simulink model "simulate_H_inf_state"  (R2013b)
settings: Solver=ode8  StartTime=0.0  StopTime=40  FixedStep=T_s  MaxStep=Auto  MinStep=Auto  RelTol=1e-3
values from neighbouring files (symbols this model uses):
  A = [0 0                                                1 0 ... (first row only)    [H_inf_state_feedback.m]    (also in Hinf_discrete_state_feedback_control (Dogan Onur ARISOY's conflicted copy 2017-02-06).m = a; Hinf_discrete_state_feedback_control.m = a; Hinf_discrete_state_feedback_control_ceyrek_tasit.m = a; bina_sistem.m = [zeros(4,4)         eye(4))
  Ac = [-1.01887           0.90506           -0.00215 ... (first row only)    [Hinf_discrete_state_feedback_control (Dogan Onur ARISOY's conflicted copy 2017-02-06).m]    (also in Hinf_discrete_state_feedback_control.m = [zeros(2) eye(2); Hinf_discrete_state_feedback_control_ceyrek_tasit.m = [0 0 1 0; LMI_Dynamic_Output.m = value(Ac); bench__lmi_state_hinf.m = [zeros(4) eye(4))
  B1 = [0;0;0;k2/m2]    [H_inf_state_feedback.m]    (also in Hinf_discrete_state_feedback_control (Dogan Onur ARISOY's conflicted copy 2017-02-06).m = b(:,1:size(Bc1,2)); Hinf_discrete_state_feedback_control.m = b(:,1:size(Bc1,2)); Hinf_discrete_state_feedback_control_ceyrek_tasit.m = b(:,1:size(Bc1,2)); bina_sistem.m = zeros(8,2))
  Bc1 = [0 ... (first row only)    [Hinf_discrete_state_feedback_control (Dogan Onur ARISOY's conflicted copy 2017-02-06).m]    (also in Hinf_discrete_state_feedback_control.m = [0;0;0;k2/m2]; Hinf_discrete_state_feedback_control_ceyrek_tasit.m = [0;0;0;k2/m2]; bench__lmi_state_hinf.m = zeros(8,2); bina__lmi_state_hinf.m = zeros(size(Ac,1),2))
  Bc2 = [1 ... (first row only)    [Hinf_discrete_state_feedback_control (Dogan Onur ARISOY's conflicted copy 2017-02-06).m]    (also in Hinf_discrete_state_feedback_control.m = [0;0;1/m1;-1/m2]; Hinf_discrete_state_feedback_control_ceyrek_tasit.m = [0;0;1/m1;-1/m2]; bench__lmi_state_hinf.m = [zeros(4,1);-1/m1;1/m2;0;0]; bina__lmi_state_hinf.m = [zeros(size(M,1),1);-1/m1;1/m2;zeros(size(M,1)-2,1)])
  C = c(1:size(Cc1,1),:)    [Hinf_discrete_state_feedback_control (Dogan Onur ARISOY's conflicted copy 2017-02-06).m]    (also in Hinf_discrete_state_feedback_control.m; Hinf_discrete_state_feedback_control_ceyrek_tasit.m; bina_sistem.m = [c1+c2          -c2              0             0; dis_state_space.m)
  Cc1 = [1  0 0 ... (first row only)    [Hinf_discrete_state_feedback_control (Dogan Onur ARISOY's conflicted copy 2017-02-06).m]    (also in Hinf_discrete_state_feedback_control.m = [1 0 0 0; Hinf_discrete_state_feedback_control_ceyrek_tasit.m = [1 0 0 0;0 1 0 0]; bench__lmi_state_hinf.m = [eye(8)]; bina__lmi_state_hinf.m = [eye(size(Ac,1))])
  E1 = b(:,size(Bc1,2)+1:size(b,2))    [Hinf_discrete_state_feedback_control (Dogan Onur ARISOY's conflicted copy 2017-02-06).m]    (also in Hinf_discrete_state_feedback_control.m; Hinf_discrete_state_feedback_control_ceyrek_tasit.m; dis_state_space.m = b(:,1:size(Bc1,2)); dynamic_output_control.mat = [0.0712527170191 0.000860589552497 4.20229137535e-06 1.11081)
  Kc = LMI_state(Ac,Bc1,Bc2,Cc1,Dc11,Dc12)    [bench__lmi_state_hinf.m]    (also in bina__lmi_state_hinf.m; dynamic_output_control.mat = [22567.2871292 -274430.071266 372104.006554 -47167.8566337 8; lmi_state_hinf.m)
  Kd = Y*Q^-1    [Hinf_discrete_state_feedback_control.m]    (also in bench__lmi_state_hinf.m = LMI_state_dis(A,B1,E1,C,B2,E2); bina__lmi_state_hinf.m = LMI_state_dis(A,B1,E1,C,B2,E2); dynamic_output_control.mat = [-308144.446712 -160117.916012 305677.057837 174380.125501 7; lmi_state_hinf.m = LMI_state_dis(A,B1,E1,C,B2,E2))
  T_s = 1e-6    (= 1e-06)    [Hinf_discrete_state_feedback_control (Dogan Onur ARISOY's conflicted copy 2017-02-06).m]    (also in Hinf_discrete_state_feedback_control.m = 0.0001; Hinf_discrete_state_feedback_control_ceyrek_tasit.m = 0.01; bench__lmi_state_hinf.m = 0.01; bina__lmi_state_hinf.m = 0.01)
settings Model: Creator=mert  LastModifiedBy=oguzhan
settings SolverCC: InitialStep=Auto
settings DebuggingCC: StateNameClashWarn=warning

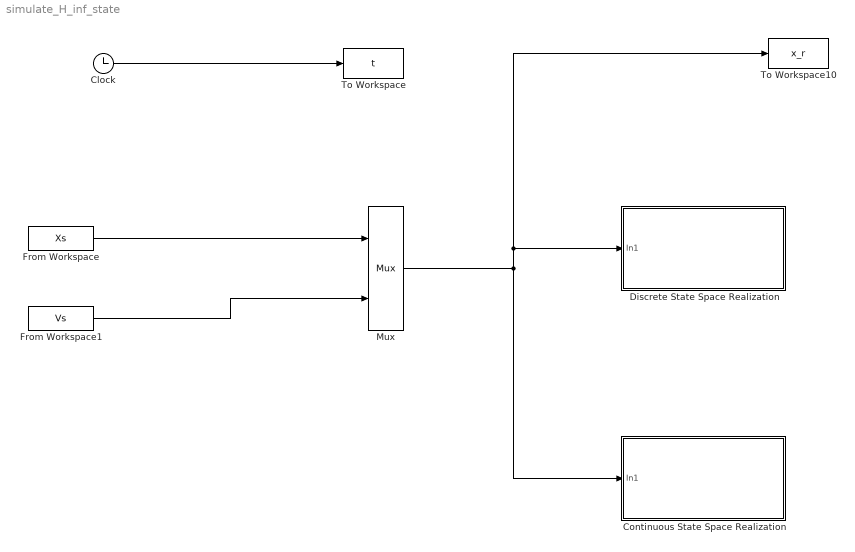
== system simulate_H_inf_state ==
  Clock : Clock
  Continuous State Space Realization : Subsystem
  Discrete State Space Realization : Subsystem
  From Workspace : FromWorkspace  VariableName=Xs
  From Workspace1 : FromWorkspace  VariableName=Vs
  Mux : Mux  Inputs=2
  To Workspace : ToWorkspace  VariableName=t  SampleTime=-1
  To Workspace10 : ToWorkspace  VariableName=x_r  SampleTime=-1
  wires:
  From Workspace/1 -> Mux/1
  From Workspace1/1 -> Mux/2
  Clock/1 -> To Workspace/1
  Mux/1 -> Continuous State Space Realization/1(In1), To Workspace10/1, Discrete State Space Realization/1(In1)

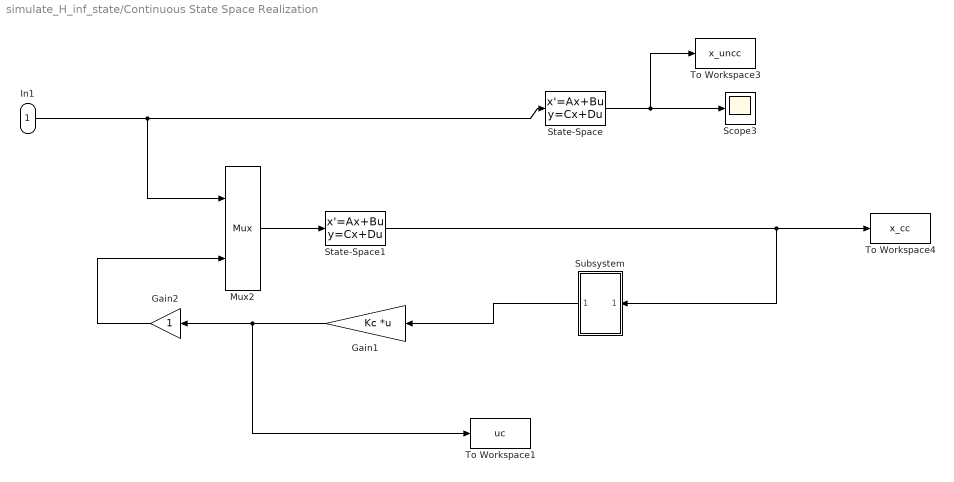
== system simulate_H_inf_state/Continuous State Space Realization ==
  In1 : Inport
  Gain1 : Gain  Gain=Kc  Multiplication=Matrix(K*u) (u vector)
  Gain2 : Gain
  Mux2 : Mux  Inputs=2
  Scope3 : Scope
      settings: SaveName=ScopeData3
  State-Space : StateSpace  A=Ac  B=Bc1  C=[Cc1;Ac(7:12,:)]  D=[zeros(size(Cc1,1),size(Bc1,2));Bc1(7:12,:)]  X0=0
  State-Space1 : StateSpace  A=Ac  B=[Bc1 Bc2]  C=[Cc1;Ac(7:12,:)]  D=[zeros(size(Cc1,1),size([Bc1 Bc2],2));[Bc1(7:12,:) Bc2(7:12,:)]]  X0=0
  Subsystem : Subsystem
  To Workspace1 : ToWorkspace  VariableName=uc  SampleTime=-1
  To Workspace3 : ToWorkspace  VariableName=x_uncc  SampleTime=-1  SaveFormat=Structure
  To Workspace4 : ToWorkspace  VariableName=x_cc  SampleTime=-1  SaveFormat=Structure
  wires:
  State-Space/1 -> To Workspace3/1, Scope3/1
  State-Space1/1 -> Subsystem/1(In1), To Workspace4/1
  Mux2/1 -> State-Space1/1
  In1/1 -> State-Space/1, Mux2/1
  Gain2/1 -> Mux2/2
  Gain1/1 -> To Workspace1/1, Gain2/1
  Subsystem/1(Out1) -> Gain1/1

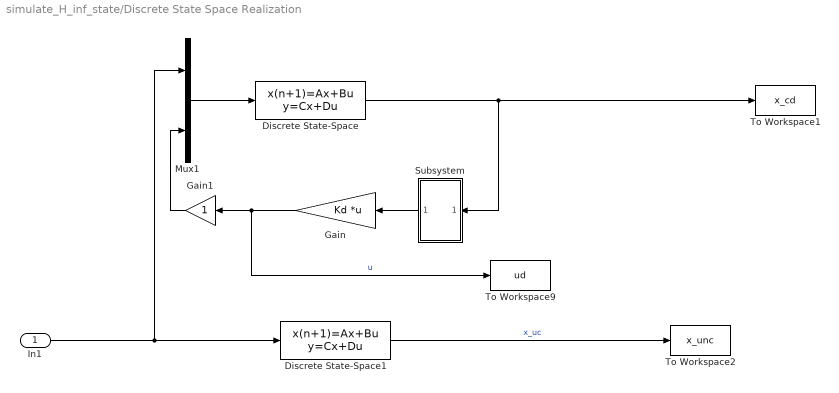
== system simulate_H_inf_state/Discrete State Space Realization ==
  In1 : Inport
  Discrete State-Space : DiscreteStateSpace  A=A  B=[E1 B1]  C=[C; A(7:12,:)]  D=[zeros(size(C,1),size([E1 B1],2));[E1(7:12,:) B1(7:12,:)]]  SampleTime=T_s
  Discrete State-Space1 : DiscreteStateSpace  A=A  B=E1  C=[C;A(7:12,:)]  D=[zeros(size(C,1),size(E1,2));E1(7:12,:)]  SampleTime=T_s
  Gain : Gain  Gain=Kd  Multiplication=Matrix(K*u) (u vector)
  Gain1 : Gain
  Mux1 : Mux  Inputs=2
  Subsystem : Subsystem
  To Workspace1 : ToWorkspace  VariableName=x_cd  SampleTime=-1  SaveFormat=Structure
  To Workspace2 : ToWorkspace  VariableName=x_unc  SampleTime=-1  SaveFormat=Structure
  To Workspace9 : ToWorkspace  VariableName=ud  SampleTime=-1
  wires:
  In1/1 -> Discrete State-Space1/1, Mux1/1
  Gain/1 -> To Workspace9/1, Gain1/1  "u"
  Discrete State-Space1/1 -> To Workspace2/1  "x_uc"
  Mux1/1 -> Discrete State-Space/1
  Discrete State-Space/1 -> To Workspace1/1, Subsystem/1(In1)
  Gain1/1 -> Mux1/2
  Subsystem/1(Out1) -> Gain/1

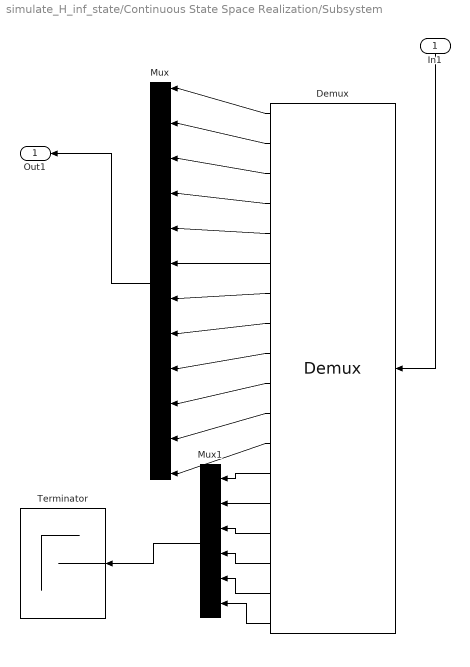
== system simulate_H_inf_state/Continuous State Space Realization/Subsystem ==
  In1 : Inport
  Demux : Demux  Outputs=18
  Mux : Mux  Inputs=12
  Mux1 : Mux  Inputs=6
  Terminator : Terminator
  Out1 : Outport
  wires:
  Mux/1 -> Out1/1
  Demux/2 -> Mux/2
  In1/1 -> Demux/1
  Demux/1 -> Mux/1
  Demux/3 -> Mux/3
  Demux/4 -> Mux/4
  Demux/5 -> Mux/5
  Demux/6 -> Mux/6
  Demux/7 -> Mux/7
  Demux/8 -> Mux/8
  Demux/9 -> Mux/9
  Demux/10 -> Mux/10
  Demux/11 -> Mux/11
  Demux/12 -> Mux/12
  Demux/13 -> Mux1/1
  Demux/14 -> Mux1/2
  Demux/15 -> Mux1/3
  Demux/16 -> Mux1/4
  Demux/17 -> Mux1/5
  Demux/18 -> Mux1/6
  Mux1/1 -> Terminator/1

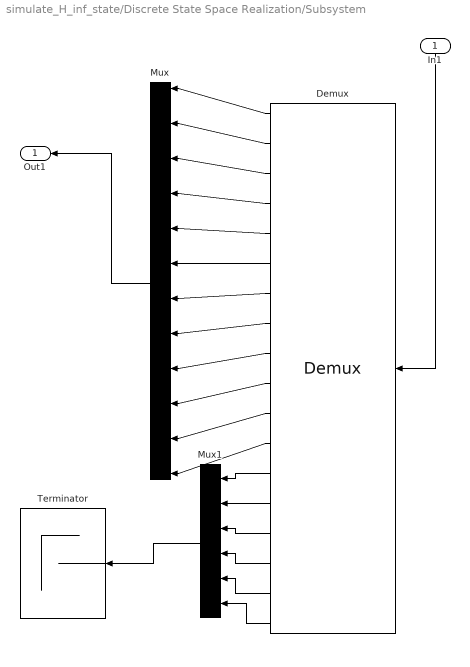
== system simulate_H_inf_state/Discrete State Space Realization/Subsystem ==
  In1 : Inport
  Demux : Demux  Outputs=18
  Mux : Mux  Inputs=12
  Mux1 : Mux  Inputs=6
  Terminator : Terminator
  Out1 : Outport
  wires:
  Mux/1 -> Out1/1
  Demux/2 -> Mux/2
  In1/1 -> Demux/1
  Demux/1 -> Mux/1
  Demux/3 -> Mux/3
  Demux/4 -> Mux/4
  Demux/5 -> Mux/5
  Demux/6 -> Mux/6
  Demux/7 -> Mux/7
  Demux/8 -> Mux/8
  Demux/9 -> Mux/9
  Demux/10 -> Mux/10
  Demux/11 -> Mux/11
  Demux/12 -> Mux/12
  Demux/13 -> Mux1/1
  Demux/14 -> Mux1/2
  Demux/15 -> Mux1/3
  Demux/16 -> Mux1/4
  Demux/17 -> Mux1/5
  Demux/18 -> Mux1/6
  Mux1/1 -> Terminator/1
